simulink model "task_1"  (R2024a)
settings: Solver=VariableStepAuto  StartTime=0.0  StopTime=20.0  RelTol=1e-3
settings Model: Creator=alexe  LastModifiedBy=alexe

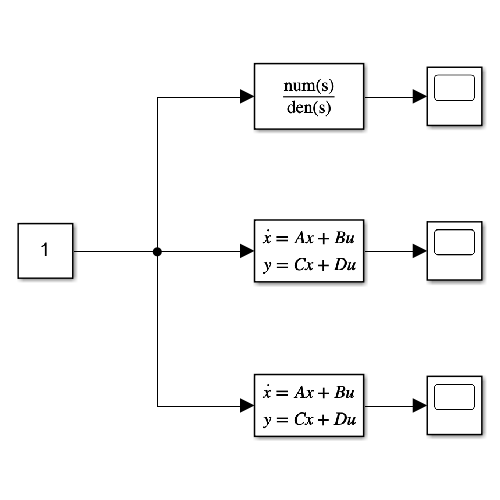
[thumbnail: Simulink's stored preview of the top-level diagram]
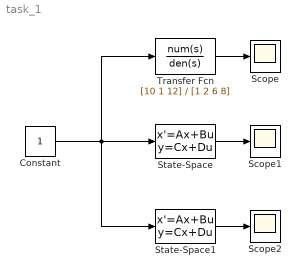
== system task_1 ==
  Constant : Constant
  Scope : Scope
  Scope1 : Scope
  Scope2 : Scope
  State-Space : StateSpace  A=[0 1 0;0 0 1;-8 -6 -2]  B=[0;0;1]  C=[12 1 10]  D=0  InitialCondition=0
  State-Space1 : StateSpace  A=[0 0 -8; 1 0 -6; 0 1 -2]  B=[12;1;10]  C=[0 0 1]  D=0  InitialCondition=0
  Transfer Fcn : TransferFcn  Numerator=[10 1 12]  Denominator=[1 2 6 8]
  wires:
  Constant/1 -> State-Space1/1, Transfer Fcn/1, State-Space/1
  Transfer Fcn/1 -> Scope/1
  State-Space/1 -> Scope1/1
  State-Space1/1 -> Scope2/1
